simulink model "DFig"  (R2024b)
settings: Solver=VariableStepAuto  StartTime=0.0  StopTime=10  RelTol=1e-3
libraries: spsThreePhaseSourceLib x1, spsWindTurbineDoublyFedInductionGeneratorPhasorTypeLib x1, sps_lib x1

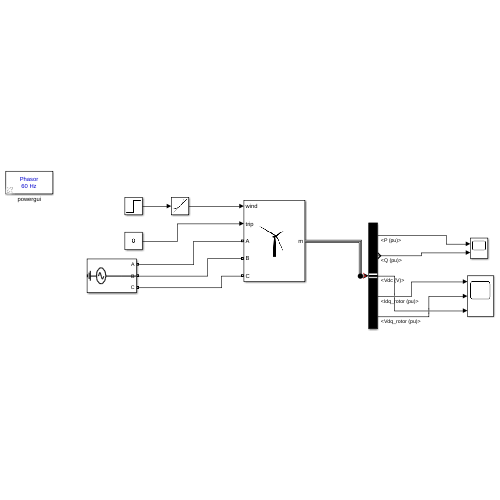
[thumbnail: Simulink's stored preview of the top-level diagram]
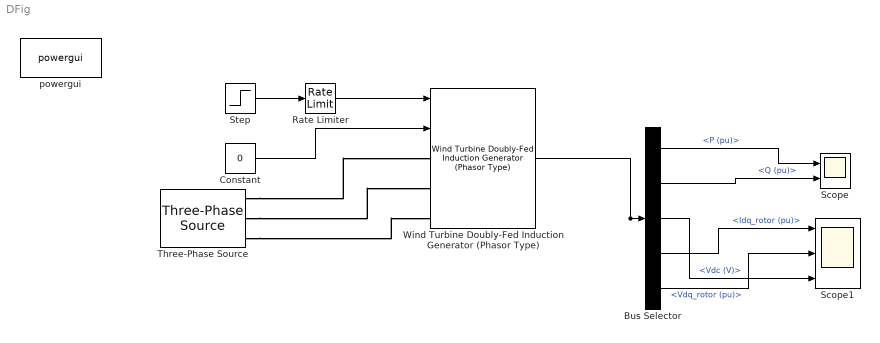
== system DFig ==
  Bus Selector : BusSelector  OutputSignals=P (pu),Q (pu),Vdc (V),Idq_rotor (pu),Vdq_rotor (pu)
  Constant : Constant  Value=0
  Rate Limiter : RateLimiter
  Scope : Scope  NumInputPorts=2
  Scope1 : Scope  NumInputPorts=3
  Step : Step  Time=4  Before=6  After=16  SampleTime=0
  Three-Phase Source : spsThreePhaseSourceLib/Three-Phase Source  InternalConnection=Yg  VoltagePhases=off  Voltage=25e3  PhaseAngle=0  Voltage_phases=[25e3 25e3 25e3]/sqrt(3)  PhaseAngles_phases=[0 -120 +120]  Frequency=60  NonIdealSource=off  SpecifyImpedance=off  ShortCircuitLevel=100e6  XRratio=7  BusType=swing  Pref=10e3  Qref=0  Prefabc=[10e3, 10e3, 10e3]  Qrefabc=[0, 0, 0]  Qmin=-inf  Qmax=inf
  Wind Turbine Doubly-Fed Induction Generator (Phasor Type) : spsWindTurbineDoublyFedInductionGeneratorPhasorTypeLib/Wind Turbine Doubly-Fed Induction Generator (Phasor Type)  ExternalTm=off  nom=[1.5e6/0.9 575 60]  sta=[ 0.00706 0.171]  rot=[ 0.005 0.156]  Lm=2.90  mec=[5.04 0.01 3]  init=[0.2 0 0 0 0 0]  speed_power=[0 0; 0.24 0.007; 0.36 0.024; 0.6 0.112; 0.96 0.46; 1.2 0.898; 1.5 0.898]  Pmec=1.5e6  speed_ABCD=[0.7 0.71 1.2 1.21]  power_C=0.73  wind_point_C=12  pitch_gain=500  pitch_max=45  pitch_rate=2  Pmax=0.5  Lchoke=[0.15 0.15/100]  init_inductor=[0 90]  Vdc_nom=1200  capacitor=10000e-6  ControlVQ=Voltage regulation  Vref=1.0  ExternalVref=off  Qref=0  ExternalQref=on  Iq_ref=0  ExternalIqref=off  Kpi_volt_reg=[1.25 300]  Xs=0.02  Kpi_Q=[0.05 5]  Kpi_power_reg=[1 100]  Kpi_dc_reg=[0.002 0.05]  Kpi_grid_side_cur_reg=[1 100]  Kpi_rotor_side_cur_reg=[0.3 8]  V_slew_rate=100  Q_slew_rate=100  power_slew_rate=1  current_slew_rate=200
      settings: LibrarySourceBlock=|
      | sps_lib/Electrical Machines/Wind Turbine
      | Doubly-Fed Induction Generator
      | (Phasor Type)
  powergui : sps_lib/powergui  Priority=1  SimulationMode=Phasor  SampleTime=50e-6  frequency=60  Iterations=50  frequencyindice=60  Pbase=100e6  ErrMax=1e-4  UnitsV=kV  UnitsW=MW  buscounter=0  FunctionMessages=off  echomessages=off  EnableUseOfTLC=off  CurrentSourceSwitches=off  DisableSnubberDevices=off  DisableRonSwitches=off  DisableVfSwitches=off  DisplayEquations=off  AutomaticDiscreteSolvers=off  SolverType=Tustin/Backward Euler (TBE)  Interpol=off  ExternalGateDelay=off  methode=off  Ts=100  x0status=blocks  SPID=on  SwTol=0  HookPort=off  NonlinearTolerance=1e-4  nMaxIteration=100  ContinueOnMaxIteration=off  RestoreLinks=warning  ResistiveCurrentMeasurement=off  Frange=[0:2:500]  Ylog=off  Xlog=on  ShowGrid=off  save=off  variable=ZData  structure=0  ZoomFFT=off  StartTime=0.0  cycles=1  DisplayStyle=1  fundamental=60  FreqAxis=off  MaxFrequency=1000  frequencyindicesteady=1  RmsSteady=1  display=off
  wires:
  Step/1 -> Rate Limiter/1
  Rate Limiter/1 -> Wind Turbine Doubly-Fed Induction Generator (Phasor Type)/1
  Constant/1 -> Wind Turbine Doubly-Fed Induction Generator (Phasor Type)/2
  Wind Turbine Doubly-Fed Induction Generator (Phasor Type)/1 -> Bus Selector/1
  Bus Selector/1 -> Scope/1  "<P (pu)>"
  Bus Selector/4 -> Scope1/1  "<Idq_rotor (pu)>"
  Bus Selector/5 -> Scope1/2  "<Vdq_rotor (pu)>"
  Bus Selector/3 -> Scope1/3  "<Vdc (V)>"
  Bus Selector/2 -> Scope/2  "<Q (pu)>"
  connections:
  Three-Phase Source/RConn1 -- Wind Turbine Doubly-Fed Induction Generator (Phasor Type)/LConn1
  Three-Phase Source/RConn2 -- Wind Turbine Doubly-Fed Induction Generator (Phasor Type)/LConn2
  Three-Phase Source/RConn3 -- Wind Turbine Doubly-Fed Induction Generator (Phasor Type)/LConn3
